simulink model "Sim_CPM_GMSK"  (R2019b)
settings: Solver=VariableStepDiscrete  StartTime=0.0  StopTime=1e5  RelTol=1e-3
libraries: commdigbbndcpm2 x8, commchan3 x4, commsink2 x4, commfilt2 x2, dspsrcs4 x2, commrandsrc3 x1, commutil2 x1
settings Model: Creator=Nuri SÖNMEZ  LastModifiedBy=Nuri SÖNMEZ
settings DataIOCC: LimitDataPoints=on  SaveOutput=off  SaveTime=off
settings OptimizationCC: BooleanDataType=off  DefaultParameterBehavior=Inlined  LocalBlockOutputs=off  LifeSpan=inf
settings DebuggingCC: AlgebraicLoopMsg=error  SingleTaskRateTransMsg=error  AllowSymbolicDim=off  SFUnexpectedBacktrackingDiag=warning  SFNoUnconditionalDefaultTransitionDiag=warning  SFExecutionAtInitializationDiag=none  ArithmeticOperatorsInVariantConditions=warning
settings SFSimCC: SimUseLocalCustomCode=off  CustomCodeUndefinedFunction=UseInterfaceOnly
settings RTWCC: RTWUseLocalCustomCode=off
settings CodeAppCC: StateflowObjectComments=on
settings GRTTargetCC: TargetLangStandard=C89/C90 (ANSI)  GeneratePreprocessorConditionals=Disable all
settings ConfigComp: CovMetricSettings=dw  CovHtmlReporting=on  CovSaveCumulativeToWorkspaceVar=on  CovSaveSingleToWorkspaceVar=on  CovExternalEMLEnable=off  CovSFcnEnable=off

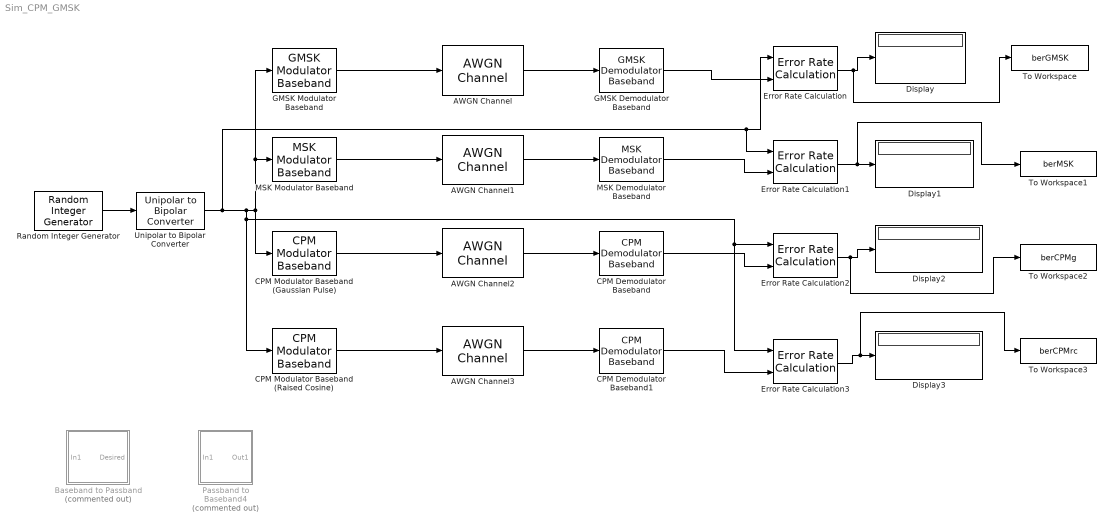
== system Sim_CPM_GMSK ==
  AWGN Channel : commchan3/AWGN Channel  InputProcessing=Columns as channels (frame based)  seed=[12345]  noiseMode="Signal to noise ratio  (Eb/No)"  EbNodB=value  EsNodB=10  SNRdB=2  bitsPerSym=1  Ps=1  Tsym=1  variance=1
      settings: SourceProductName=Communications Toolbox
  AWGN Channel1 : commchan3/AWGN Channel  InputProcessing=Columns as channels (frame based)  seed=[12345]  noiseMode="Signal to noise ratio  (Eb/No)"  EbNodB=value  EsNodB=10  SNRdB=0  bitsPerSym=1  Ps=1  Tsym=1  variance=1
      settings: SourceProductName=Communications Toolbox
  AWGN Channel2 : commchan3/AWGN Channel  InputProcessing=Columns as channels (frame based)  seed=[12345]  noiseMode="Signal to noise ratio  (Eb/No)"  EbNodB=value  EsNodB=10  SNRdB=0  bitsPerSym=1  Ps=1  Tsym=1  variance=1
      settings: SourceProductName=Communications Toolbox
  AWGN Channel3 : commchan3/AWGN Channel  InputProcessing=Columns as channels (frame based)  seed=[12345]  noiseMode="Signal to noise ratio  (Eb/No)"  EbNodB=value  EsNodB=10  SNRdB=0  bitsPerSym=1  Ps=1  Tsym=1  variance=1
      settings: SourceProductName=Communications Toolbox
  Baseband to Passband : Subsystem  Commented=on
  CPM Demodulator Baseband : commdigbbndcpm2/CPM Demodulator Baseband  Mnum=2  outputType=Integer  mappingType=Binary  modIdx=0.5  pulseShape=Gaussian  BT=0.25  mainLobePulseLength=1  rollOff=0.2  pulseLength=1  preHistory=1  phaseOffset=0  samplesPerSymbol=8  RateOptions=Enforce single-rate processing  traceBack=16  outDType=double
      settings: SourceProductName=Communications Toolbox  SourceProductBaseCode=CM
  CPM Demodulator Baseband1 : commdigbbndcpm2/CPM Demodulator Baseband  Mnum=2  outputType=Integer  mappingType=Binary  modIdx=0.5  pulseShape=Raised Cosine  BT=0.3  mainLobePulseLength=1  rollOff=0.2  pulseLength=1  preHistory=1  phaseOffset=0  samplesPerSymbol=8  RateOptions=Enforce single-rate processing  traceBack=16  outDType=double
      settings: SourceProductName=Communications Toolbox  SourceProductBaseCode=CM
  CPM Modulator Baseband (Gaussian Pulse) : commdigbbndcpm2/CPM Modulator Baseband  Mnum=2  inputType=Integer  mappingType=Binary  modIdx=0.5  pulseShape=Gaussian  BT=0.25  mainLobePulseLength=1  rollOff=0.2  pulseLength=1  preHistory=1  phaseOffset=0  samplesPerSymbol=8  RateOptions=Enforce single-rate processing  outDataType=double
      settings: SourceProductName=Communications Toolbox  SourceProductBaseCode=CM
  CPM Modulator Baseband (Raised Cosine) : commdigbbndcpm2/CPM Modulator Baseband  Mnum=2  inputType=Integer  mappingType=Binary  modIdx=0.5  pulseShape=Raised Cosine  BT=0.3  mainLobePulseLength=1  rollOff=0.2  pulseLength=1  preHistory=1  phaseOffset=0  samplesPerSymbol=8  RateOptions=Enforce single-rate processing  outDataType=double
      settings: SourceProductName=Communications Toolbox  SourceProductBaseCode=CM
  Display{,1..3} (4 alike) : Display
  Error Rate Calculation{,1..3} (4 alike) : commsink2/Error Rate Calculation  N=16  st_delay=0  cp_mode=Entire frame  subframe=[]  PMode=Port  WsName=ErrorVec  RsMode2=off  stop=off  numErr=100  maxBits=1e6
      settings: SourceProductName=Communications Toolbox
  GMSK Demodulator Baseband : commdigbbndcpm2/GMSK Demodulator Baseband  OutputType=Integer  BT=.25  pulseLength=1  preHistory=1  phaseOffset=0  samplesPerSymbol=8  RateOptions=Enforce single-rate processing  traceBack=16  outDType=double
      settings: SourceProductName=Communications Toolbox  SourceProductBaseCode=CM
  GMSK Modulator Baseband : commdigbbndcpm2/GMSK Modulator Baseband  inputType=Integer  BT=.25  pulseLength=1  preHistory=1  phaseOffset=0  samplesPerSymbol=8  RateOptions=Enforce single-rate processing  outDataType=double
      settings: SourceProductName=Communications Toolbox  SourceProductBaseCode=CM
  MSK Demodulator Baseband : commdigbbndcpm2/MSK Demodulator Baseband  outputType=Integer  phaseOffset=0  samplesPerSymbol=8  RateOptions=Enforce single-rate processing  traceBack=16  outDType=double
      settings: SourceProductName=Communications Toolbox  SourceProductBaseCode=CM
  MSK Modulator Baseband : commdigbbndcpm2/MSK Modulator Baseband  inputType=Integer  phaseOffset=0  samplesPerSymbol=8  RateOptions=Enforce single-rate processing  outDataType=double
      settings: SourceProductName=Communications Toolbox  SourceProductBaseCode=CM
  Passband to Baseband4 : Subsystem  Commented=on
  Random Integer Generator : commrandsrc3/Random Integer Generator  SetSize=2  SeedSource=Parameter  Seed=[12345]  SampleTime=1  SamplesPerFrame=100  OutputDataType=double  SimulateUsing=Interpreted execution
      settings: SourceProductName=Communications Toolbox
  To Workspace : ToWorkspace  VariableName=berGMSK  SampleTime=-1
      settings: Save2DSignal=2-D array (concatenate along first dimension)
  To Workspace1 : ToWorkspace  VariableName=berMSK  SampleTime=-1
      settings: Save2DSignal=2-D array (concatenate along first dimension)
  To Workspace2 : ToWorkspace  VariableName=berCPMg  SampleTime=-1
      settings: Save2DSignal=2-D array (concatenate along first dimension)
  To Workspace3 : ToWorkspace  VariableName=berCPMrc  SampleTime=-1
      settings: Save2DSignal=2-D array (concatenate along first dimension)
  Unipolar to Bipolar Converter : commutil2/Unipolar to Bipolar Converter  M=2  polarity=Positive  dataType=Inherit via internal rule
      settings: SourceProductName=Communications Toolbox
  wires:
  Random Integer Generator/1 -> Unipolar to Bipolar Converter/1
  Unipolar to Bipolar Converter/1 -> Error Rate Calculation3/1, Error Rate Calculation2/1, CPM Modulator Baseband (Raised Cosine)/1, CPM Modulator Baseband (Gaussian Pulse)/1, MSK Modulator Baseband/1, GMSK Modulator Baseband/1, Error Rate Calculation1/1, Error Rate Calculation/1
  CPM Demodulator Baseband1/1 -> Error Rate Calculation3/2
  CPM Demodulator Baseband/1 -> Error Rate Calculation2/2
  MSK Demodulator Baseband/1 -> Error Rate Calculation1/2
  GMSK Demodulator Baseband/1 -> Error Rate Calculation/2
  Error Rate Calculation/1 -> To Workspace/1, Display/1
  Error Rate Calculation1/1 -> To Workspace1/1, Display1/1
  Error Rate Calculation2/1 -> To Workspace2/1, Display2/1
  Error Rate Calculation3/1 -> To Workspace3/1, Display3/1
  AWGN Channel/1 -> GMSK Demodulator Baseband/1
  AWGN Channel1/1 -> MSK Demodulator Baseband/1
  MSK Modulator Baseband/1 -> AWGN Channel1/1
  AWGN Channel2/1 -> CPM Demodulator Baseband/1
  CPM Modulator Baseband (Gaussian Pulse)/1 -> AWGN Channel2/1
  AWGN Channel3/1 -> CPM Demodulator Baseband1/1
  CPM Modulator Baseband (Raised Cosine)/1 -> AWGN Channel3/1
  GMSK Modulator Baseband/1 -> AWGN Channel/1

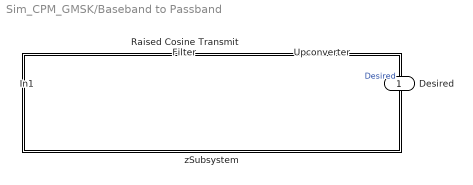
== system Sim_CPM_GMSK/Baseband to Passband ==
  In1 : Inport
  Raised Cosine Transmit Filter : commfilt2/Raised Cosine Transmit Filter  filtType=Square root  R=0.2  filtSpan=8  N=8  filterGain=1  InputProcessing=Columns as channels (frame based)  RateOptions=Enforce single-rate processing  framing=Mute  checkCoeff=off  variableName=rcTxFilt1  checkGain=Normalized  sampMode=Mute  saveAsFlag=0  currentFiltSpan=2*(4)  D=4  launchFVT=off  roundingMode=Floor  overflowMode=off  coeffDataTypeStr=Inherit: Same word length as input  coeffMin=[]  coeffMax=[]  coeffLastDataTypeStr=Inherit: Same word length as input  outputDataTypeStr=Inherit: Same as accumulator  outputMin=[]  outputMax=[]  outputLastDataTypeStr=Inherit: Same as accumulator
      settings: SourceProductName=Communications Toolbox
  Upconverter : Subsystem
      mask Display: disp('Upconverter')
  zSubsystem : Subsystem
      mask Display: disp('')
  Desired : Outport
  wires:
  In1/1 -> Raised Cosine Transmit Filter/1
  Upconverter/1(Out) -> Desired/1  "Desired"
  Raised Cosine Transmit Filter/1 -> Upconverter/1(In)

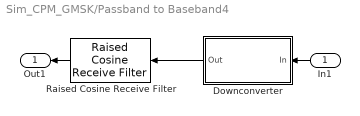
== system Sim_CPM_GMSK/Passband to Baseband4 ==
  In1 : Inport
  Downconverter : Subsystem
      mask Display: disp('Downconverter')
  Raised Cosine Receive Filter : commfilt2/Raised Cosine Receive Filter  filtType=Square root  R=0.2  filtSpan=8  N=8  downFactor=8  downOffset=0  filterGain=2  InputProcessing=Columns as channels (frame based)  RateOptions=Enforce single-rate processing  framing=Mute  checkCoeff=off  variableName=rcRxFilt1  currentFiltSpan=2*(4)  D=4  inputOffset=0  sampMode=Mute  saveAsFlag=0  rateMode=Downsampling  checkGain=User-specified  launchFVT=off  roundingMode=Floor  overflowMode=off  coeffDataTypeStr=Inherit: Same word length as input  coeffMin=[]  coeffMax=[]  coeffLastDataTypeStr=Inherit: Same word length as input  accumDataTypeStr=Inherit: Same as product output  accumLastDataTypeStr=Inherit: Same as product output  outputDataTypeStr=Inherit: Same as accumulator  outputMin=[]  outputMax=[]  outputLastDataTypeStr=Inherit: Same as accumulator
      settings: SourceProductName=Communications Toolbox
  Out1 : Outport
  wires:
  Downconverter/1(Out) -> Raised Cosine Receive Filter/1
  Raised Cosine Receive Filter/1 -> Out1/1
  In1/1 -> Downconverter/1(In)

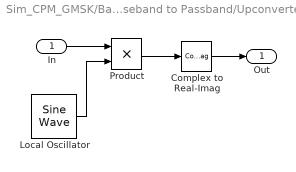
== system Sim_CPM_GMSK/Baseband to Passband/Upconverter ==
  In : Inport
  Complex to Real-Imag : ComplexToRealImag  Output=Real
  Local Oscillator : dspsrcs4/Sine Wave  Amplitude=1  Frequency=8.5e8  Phase=0  SampleMode=Discrete  OutComplex=Complex  CompMethod=Trigonometric fcn  TableSize=Speed  SampleTime=(1e-6) /8  SamplesPerFrame=800  ResetState=Restart at time zero  OutputFrames=off  dataType=double  wordLen=16  udDataType=sfix(16)  fracBitsMode=Best precision  numFracBits=15  OutDataTypeStr=double  LastOutDataTypeStr=double
  Product : Product  RndMeth=Zero
  Out : Outport  VectorParamsAs1DForOutWhenUnconnected=off
  wires:
  Complex to Real-Imag/1 -> Out/1
  Product/1 -> Complex to Real-Imag/1
  Local Oscillator/1 -> Product/2
  In/1 -> Product/1

== system Sim_CPM_GMSK/Baseband to Passband/zSubsystem ==

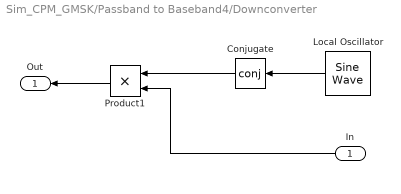
== system Sim_CPM_GMSK/Passband to Baseband4/Downconverter ==
  In : Inport
  Conjugate : Math  Operator=conj  SaturateOnIntegerOverflow=on
  Local Oscillator : dspsrcs4/Sine Wave  Amplitude=1  Frequency=8.5e8  Phase=0  SampleMode=Discrete  OutComplex=Complex  CompMethod=Trigonometric fcn  TableSize=Speed  SampleTime=(1e-6) /8  SamplesPerFrame=800  ResetState=Restart at time zero  OutputFrames=off  dataType=double  wordLen=16  udDataType=sfix(16)  fracBitsMode=Best precision  numFracBits=15  OutDataTypeStr=double  LastOutDataTypeStr=double
  Product1 : Product  RndMeth=Zero
  Out : Outport  VectorParamsAs1DForOutWhenUnconnected=off
  wires:
  Conjugate/1 -> Product1/1
  Product1/1 -> Out/1
  In/1 -> Product1/2
  Local Oscillator/1 -> Conjugate/1
